simulink model "project_2023_12_25_P121"  (R2017b)
settings: Solver=ode5  StartTime=0.0  StopTime=500  FixedStep=0.1  RelTol=1e-3
libraries: simulink x1
settings Model: Creator=Administrator  LastModifiedBy=Administrator

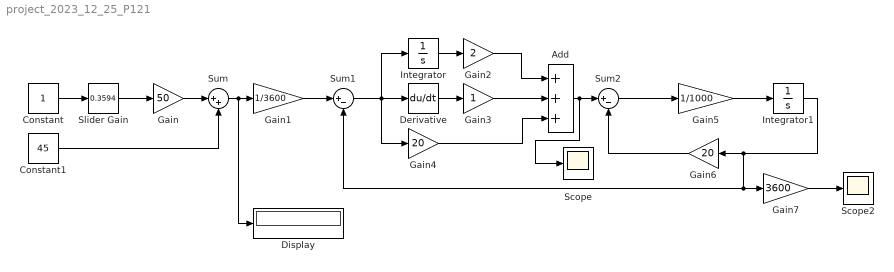
== system project_2023_12_25_P121 ==
  Add : Sum  Inputs=+++
  Constant : Constant
  Constant1 : Constant  Value=45
  Derivative : Derivative
  Display : Display
  Gain : Gain  Gain=50
  Gain1 : Gain  Gain=1/3600
  Gain2 : Gain  Gain=2
  Gain3 : Gain
  Gain4 : Gain  Gain=20
  Gain5 : Gain  Gain=1/1000
  Gain6 : Gain  Gain=20
  Gain7 : Gain  Gain=3600
  Integrator : Integrator
  Integrator1 : Integrator
  Scope : Scope
  Scope2 : Scope
  Slider Gain : simulink/Math Operations/Slider Gain  gain=0.3594  low=0  high=2
  Sum : Sum  Inputs=|++
  Sum1 : Sum  Inputs=|+-
  Sum2 : Sum  Inputs=|+-
  wires:
  Sum/1 -> Display/1, Gain1/1
  Add/1 -> Scope/1, Sum2/1
  Gain5/1 -> Integrator1/1
  Gain7/1 -> Scope2/1
  Constant/1 -> Slider Gain/1
  Slider Gain/1 -> Gain/1
  Gain/1 -> Sum/1
  Constant1/1 -> Sum/2
  Gain1/1 -> Sum1/1
  Sum1/1 -> Gain4/1, Derivative/1, Integrator/1
  Integrator/1 -> Gain2/1
  Derivative/1 -> Gain3/1
  Gain3/1 -> Add/2
  Gain2/1 -> Add/1
  Gain4/1 -> Add/3
  Sum2/1 -> Gain5/1
  Integrator1/1 -> Sum1/2, Gain7/1, Gain6/1
  Gain6/1 -> Sum2/2
